simulink library "gliderCtrl_cl"  (R2022a)
settings: Solver=VariableStepAuto  StartTime=0.0  StopTime=10.0  RelTol=1e-3
undefined symbols (not defined in the file or in its folder): initializeBussesFromBlock
settings Model: Creator=mitch  LastModifiedBy=lhill8
settings SolverCC: AlgebraicLoopSolver=TrustRegion
settings DebuggingCC: UnconnectedInputMsg=warning  UnconnectedOutputMsg=warning  UnconnectedLineMsg=warning  SFMachineParentedDataDiag=warning

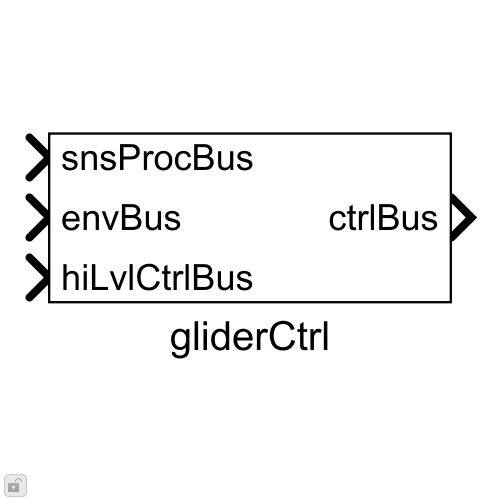
[thumbnail: Simulink's stored preview of the top-level diagram]
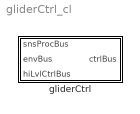
== system gliderCtrl_cl ==
  gliderCtrl : Subsystem  LoadFcn=initializeBussesFromBlock(gcb)  InitFcn=initializeBussesFromBlock(gcb)  StartFcn=initializeBussesFromBlock(gcb)

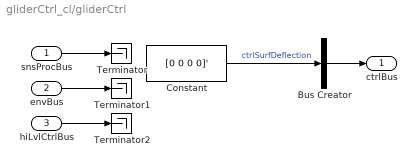
== system gliderCtrl_cl/gliderCtrl ==
  snsProcBus : Inport  OutDataTypeStr=Bus: sensorsProcessingBus
  envBus : Inport  Port=2  OutDataTypeStr=Bus: envBus
  hiLvlCtrlBus : Inport  Port=3  OutDataTypeStr=Bus: hiLvlCtrlBus
  Bus Creator : BusCreator  Inputs=1  OutDataTypeStr=Bus: gndStnCtrlBus  NonVirtualBus=on
  Constant : Constant  Value=[0 0 0 0]'
  Terminator : Terminator
  Terminator1 : Terminator
  Terminator2 : Terminator
  ctrlBus : Outport  OutDataTypeStr=Bus: gndStnCtrlBus  VectorParamsAs1DForOutWhenUnconnected=off
  wires:
  envBus/1 -> Terminator1/1
  hiLvlCtrlBus/1 -> Terminator2/1
  Bus Creator/1 -> ctrlBus/1
  Constant/1 -> Bus Creator/1  "ctrlSurfDeflection"
  snsProcBus/1 -> Terminator/1
